simulink library "mylibrary"  (Simulink 7.7)
settings: Solver=ode45  StartTime=0.0  StopTime=10.0  RelTol=1e-3
settings Model: Creator=hnine  LastModifiedBy=hnine

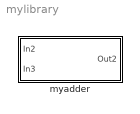
== system mylibrary ==
  myadder : Subsystem

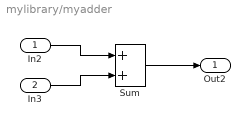
== system mylibrary/myadder ==
  In2 : Inport
  In3 : Inport  Port=2
  Sum : Sum
  Out2 : Outport
  wires:
  Sum/1 -> Out2/1
  In2/1 -> Sum/1
  In3/1 -> Sum/2
